simulink model "HL_control_pos_FFforce_RC_WirtualWall_Sync"  (R2020a)
settings: Solver=ode4  StartTime=0.0  StopTime=inf  FixedStep=0.001  RelTol=1e-3
libraries: xpcethercatlib x42, simulink x12, slrtlib x10, AssistOn_Gait_Lib x6
(part 2 of 3)

== system HL_control_pos_FFforce_RC_WirtualWall_Sync/Plot//Record Outputs/Left leg readings ==
  L outs : Inport
  Bus Creator : BusCreator  Inputs=2
  Bus Creator1 : BusCreator  Inputs=2
  Bus Creator2 : BusCreator  Inputs=2
  Bus Selector1 : BusSelector  OutputSignals=left.pos.y,left.vel.vy,left.force.Fy  OutputAsBus=on
  Bus Selector2 : BusSelector  OutputSignals=left.pos.theta,left.vel.omega,left.force.Tz  OutputAsBus=on
  Bus Selector4 : BusSelector  OutputSignals=left.pos.x,left.vel.vx,left.force.Fx  OutputAsBus=on
  Bus Selector5 : BusSelector  OutputSignals=lpos.lx,lvel.lvx,lFT.lFx  OutputAsBus=on
  Bus Selector6 : BusSelector  OutputSignals=lpos.ly,lvel.lvy,lFT.lFy  OutputAsBus=on
  Bus Selector7 : BusSelector  OutputSignals=lpos.ltheta,lvel.lomega,lFT.lTz  OutputAsBus=on
  "Scope " : slrtlib/Displays and Logging/Scope   scopeno=4  scopetype=Target  autostart=on  viewmode=Graphical sliding  formatstr='%15.6f'  grid=on  ylimits=80*[-1, 1]  nosamples=500  noprepostsamples=0  interleave=20  triggermode=FreeRun  triggersignal=1  trigsignalfromport=off  triggerlevel=0.0  triggerslope=Either  triggerscope=1  triggersample=0  filename=data.dat  mode=Lazy  writesize=512  autorestart=off  dynamicfilemode=off  maxwritefilesize=512*1024^2
  Scope 1 : slrtlib/Displays and Logging/Scope   scopeno=5  scopetype=Target  autostart=on  viewmode=Graphical sliding  formatstr='%15.6f'  grid=on  ylimits=80*[-1, 1]  nosamples=500  noprepostsamples=0  interleave=20  triggermode=FreeRun  triggersignal=1  trigsignalfromport=off  triggerlevel=0.0  triggerslope=Either  triggerscope=1  triggersample=0  filename=data.dat  mode=Lazy  writesize=512  autorestart=off  dynamicfilemode=off  maxwritefilesize=512*1024^2
  Scope 2 : slrtlib/Displays and Logging/Scope   scopeno=6  scopetype=Target  autostart=on  viewmode=Graphical rolling  formatstr='%15.6f'  grid=on  ylimits=pi/2*[-1, 1]  nosamples=500  noprepostsamples=0  interleave=20  triggermode=FreeRun  triggersignal=1  trigsignalfromport=off  triggerlevel=0.0  triggerslope=Either  triggerscope=1  triggersample=0  filename=data.dat  mode=Lazy  writesize=512  autorestart=off  dynamicfilemode=off  maxwritefilesize=512*1024^2
  Subsystem : Subsystem  Commented=on
  wires:
  Bus Creator/1 -> "Scope "/1
  [Ref] -> Bus Selector2/1, Bus Selector1/1, Bus Selector4/1
  Bus Creator1/1 -> Scope 1/1
  Bus Selector1/1 -> Bus Creator1/1
  Bus Selector6/1 -> Bus Creator1/2
  Bus Selector4/1 -> Bus Creator/1
  L outs/1 -> Bus Selector5/1, Bus Selector6/1, Bus Selector7/1
  Bus Creator2/1 -> Scope 2/1
  Bus Selector5/1 -> Bus Creator/2
  Bus Selector7/1 -> Bus Creator2/2
  Bus Selector2/1 -> Bus Creator2/1

== system HL_control_pos_FFforce_RC_WirtualWall_Sync/Plot//Record Outputs/Right leg readings ==
  R outs : Inport
  Bus Creator1 : BusCreator  Inputs=2
  Bus Creator2 : BusCreator  Inputs=2
  Bus Creator3 : BusCreator  Inputs=2
  Bus Selector1 : BusSelector  OutputSignals=right.pos.y,right.vel.vy,right.force.Fy  OutputAsBus=on
  Bus Selector2 : BusSelector  OutputSignals=right.pos.x,right.vel.vx,right.force.Fx  OutputAsBus=on
  Bus Selector3 : BusSelector  OutputSignals=rpos.rx,rvel.rvx,rFT.rFx  OutputAsBus=on
  Bus Selector4 : BusSelector  OutputSignals=rpos.ry,rvel.rvy,rFT.rFy  OutputAsBus=on
  Bus Selector6 : BusSelector  OutputSignals=rpos.rtheta,rvel.romega,rFT.rTz  OutputAsBus=on
  Bus Selector7 : BusSelector  OutputSignals=right.pos.theta,right.vel.omega,right.force.Tz  OutputAsBus=on
  Scope 1 : slrtlib/Displays and Logging/Scope   scopeno=2  scopetype=Target  autostart=on  viewmode=Graphical sliding  formatstr='%15.6f'  grid=on  ylimits=80*[-1, 1]  nosamples=500  noprepostsamples=0  interleave=20  triggermode=FreeRun  triggersignal=1  trigsignalfromport=off  triggerlevel=0.0  triggerslope=Either  triggerscope=1  triggersample=0  filename=rhipinc.dat  mode=Lazy  writesize=512  autorestart=off  dynamicfilemode=off  maxwritefilesize=512*1024^2
  Scope 2 : slrtlib/Displays and Logging/Scope   scopeno=1  scopetype=Target  autostart=on  viewmode=Graphical rolling  formatstr='%15.6f'  grid=on  ylimits=80*[-1, 1]  nosamples=500  noprepostsamples=0  interleave=20  triggermode=FreeRun  triggersignal=1  trigsignalfromport=off  triggerlevel=0.0  triggerslope=Either  triggerscope=1  triggersample=0  filename=rhipinc.dat  mode=Lazy  writesize=512  autorestart=off  dynamicfilemode=off  maxwritefilesize=512*1024^2
  Scope 5 : slrtlib/Displays and Logging/Scope   scopeno=3  scopetype=Target  autostart=on  viewmode=Graphical rolling  formatstr='%15.6f'  grid=on  ylimits=pi/2*[-1, 1]  nosamples=500  noprepostsamples=0  interleave=20  triggermode=FreeRun  triggersignal=1  trigsignalfromport=off  triggerlevel=0.0  triggerslope=Either  triggerscope=1  triggersample=0  filename=rhipinc.dat  mode=Lazy  writesize=512  autorestart=off  dynamicfilemode=off  maxwritefilesize=512*1024^2
  Subsystem : Subsystem  Commented=on
  wires:
  Bus Creator1/1 -> Scope 1/1
  Bus Creator2/1 -> Scope 5/1
  Bus Selector2/1 -> Bus Creator3/1
  R outs/1 -> Bus Selector3/1, Bus Selector4/1, Bus Selector6/1
  Bus Creator3/1 -> Scope 2/1
  Bus Selector4/1 -> Bus Creator1/2
  Bus Selector1/1 -> Bus Creator1/1
  Bus Selector6/1 -> Bus Creator2/2
  [Ref] -> Bus Selector7/1, Bus Selector1/1, Bus Selector2/1
  Bus Selector3/1 -> Bus Creator3/2
  Bus Selector7/1 -> Bus Creator2/1

== system HL_control_pos_FFforce_RC_WirtualWall_Sync/Right Leg/Jacobian Transpose [mN] -> [mN.mm//rad] ==
  states : Inport
  force [mN] : Inport  Port=2
  Bus Selector1 : BusSelector  OutputSignals=R disk mot.disk angle,R pos.s1s2s3,R pos.xytheta  OutputAsBus=on
  Bus to Vector : BusToVector
  S-Function : S-Function  FunctionName=RRP_Jacobian_Transpose  SFunctionModules='RRP_Jacobian_Transpose_wrapper'  SFunctionDeploymentMode=off  EnableBusSupport=off
  torque [mN.mm/rad] : Outport
  wires:
  S-Function/1 -> torque [mN.mm/rad]/1
  force [mN]/1 -> S-Function/2
  states/1 -> Bus Selector1/1
  Bus Selector1/1 -> Bus to Vector/1
  Bus to Vector/1 -> S-Function/1

== system HL_control_pos_FFforce_RC_WirtualWall_Sync/Right Leg/Position Controller -> [mN] ==
  ref pos : Inport
  ref vel : Inport  Port=2
  estimated out : Inport  Port=3
  " " : Sum
  Bus Selector : BusSelector  OutputSignals=R pos.xytheta,R vel
  D_Controller : Subsystem
  "P_Controller\t" : Subsystem
  Control Force : Outport
  wires:
  Bus Selector/2 -> D_Controller/1(Act_Vel)  "<R vel>"
  estimated out/1 -> Bus Selector/1
  "P_Controller\t"/1(P control out) -> " "/1
  Bus Selector/1 -> "P_Controller\t"/2(Act_Pos)  "<xytheta>"
  " "/1 -> Control Force/1  "Control Force"
  D_Controller/1(D control out) -> " "/2
  ref vel/1 -> D_Controller/2(Ref_vel)
  ref pos/1 -> "P_Controller\t"/1(Ref_Pos)

== system HL_control_pos_FFforce_RC_WirtualWall_Sync/Right Leg/R Actuation ==
  torque [mN.mm/rad] : Inport
  M1 Target Torque : xpcethercatlib/EtherCAT PDO Transmit   Priority=3  sig_name=M1 (MAXPOS).CST Mode.CST Outputs.TargetTorque  sig_offset=848  sig_type=int16  type_size=16  sig_dim=1  device_id=0  sample_time=0.001000
      settings: SourceProductBaseCode=XP
  M2 Target Torque : xpcethercatlib/EtherCAT PDO Transmit   Priority=3  sig_name=M2 (MAXPOS).CST Mode.CST Outputs.TargetTorque  sig_offset=992  sig_type=int16  type_size=16  sig_dim=1  device_id=0  sample_time=0.001000
      settings: SourceProductBaseCode=XP
  M3 Target Torque : xpcethercatlib/EtherCAT PDO Transmit   Priority=3  sig_name=M3 (MAXPOS).CST Mode.CST Outputs.TargetTorque  sig_offset=1104  sig_type=int16  type_size=16  sig_dim=1  device_id=0  sample_time=0.001000
      settings: SourceProductBaseCode=XP
  Target Torque : Subsystem
  wires:
  torque [mN.mm/rad]/1 -> Target Torque/1(torque)
  Target Torque/1(M1_torque) -> M1 Target Torque/1
  Target Torque/2(M2_torque) -> M2 Target Torque/1
  Target Torque/3(M3_torque) -> M3 Target Torque/1

== system HL_control_pos_FFforce_RC_WirtualWall_Sync/Right Leg/R Outputs ==
  3RRP Forward Kinematics : AssistOn_Gait_Lib/3RRP Forward Kinematics  SystemSampleTime=-1  Latency=0  AutoFrameSizeCalculation=off
  3RRP Motion Level Kinematics : AssistOn_Gait_Lib/3RRP Motion Level Kinematics  SystemSampleTime=-1  Latency=0  AutoFrameSizeCalculation=off
  Bus Creator : BusCreator  Inputs=7
  Bus Selector1 : BusSelector  OutputSignals=disk angle
  R 3RRP : AssistOn_Gait_Lib/3RRP  SystemSampleTime=-1  Latency=0  AutoFrameSizeCalculation=off
      link override 3RRP Motor Encoder Increments/M1 Position Value: sig_name=M1 (MAXPOS).CST Mode.CST Inputs.PositionActualValue  sig_offset=848  sig_type=int32  type_size=32  sig_dim=1
      link override 3RRP Motor Encoder Increments/M2 Position Value: sig_name=M2 (MAXPOS).CST Mode.CST Inputs.PositionActualValue  sig_offset=992  sig_type=int32  type_size=32  sig_dim=1
      link override 3RRP Motor Encoder Increments/M3 Position Value: sig_name=M3 (MAXPOS).CST Mode.CST Inputs.PositionActualValue  sig_offset=1104  sig_type=int32  type_size=32  sig_dim=1
      link override 3RRP Motor Torque Readings/M1 Velocity Value: sig_name=M1 (MAXPOS).CST Mode.CST Inputs.TorqueActualValue  sig_offset=912  sig_type=int16  type_size=16  sig_dim=1
      link override 3RRP Motor Torque Readings/M2 Velocity Value: sig_name=M2 (MAXPOS).CST Mode.CST Inputs.TorqueActualValue  sig_offset=1056  sig_type=int16  type_size=16  sig_dim=1
      link override 3RRP Motor Torque Readings/M3 Velocity Value: sig_name=M3 (MAXPOS).CST Mode.CST Inputs.TorqueActualValue  sig_offset=1168  sig_type=int16  type_size=16  sig_dim=1
      link override 3RRP Motor Velocity Readings/M1 Velocity Value: sig_name=M1 (MAXPOS).CST Mode.CST Inputs.Velocity Actual Value Averaged  sig_offset=880  sig_type=int32  type_size=32  sig_dim=1
      link override 3RRP Motor Velocity Readings/M2 Velocity Value: sig_name=M2 (MAXPOS).CST Mode.CST Inputs.Velocity Actual Value Averaged  sig_offset=1024  sig_type=int32  type_size=32  sig_dim=1
      link override 3RRP Motor Velocity Readings/M3 Velocity Value: sig_name=M3 (MAXPOS).CST Mode.CST Inputs.Velocity Actual Value Averaged  sig_offset=1136  sig_type=int32  type_size=32  sig_dim=1
  R Foot : Subsystem
  R Thigh : Subsystem
  R leg outs : Outport
  wires:
  R 3RRP/2 -> 3RRP Motion Level Kinematics/2, Bus Creator/5, Bus Selector1/1  "R disk mot"
  R Foot/1(Foot sens R) -> Bus Creator/7  "R_foot_sens"
  Bus Creator/1 -> R leg outs/1
  3RRP Forward Kinematics/1 -> 3RRP Motion Level Kinematics/1, Bus Creator/3  "R pos"
  Bus Selector1/1 -> 3RRP Forward Kinematics/1  "<disk angle>"
  3RRP Motion Level Kinematics/1 -> Bus Creator/4  "R vel"
  R Thigh/1(FT vals) -> Bus Creator/6  "R_thigh_FT"
  R 3RRP/1 -> Bus Creator/2  "R disk torque"
  [R_motor_T_demands] -> Bus Creator/1

== system HL_control_pos_FFforce_RC_WirtualWall_Sync/Right Leg/Velocity Sourced Compansator ==
  Velocity Disks : Inport
  Mode : Inport  Port=2
  DiskGains : Constant  Value=[1;1;3]
  MATLAB Function1 : MATLAB Function  TreatAsAtomicUnit=on
  Disk Forces : Outport
  wires:
  Velocity Disks/1 -> MATLAB Function1/1(Vel)
  Mode/1 -> MATLAB Function1/3(Mode)
  DiskGains/1 -> MATLAB Function1/2(MaxGain)
  MATLAB Function1/1(Torque) -> Disk Forces/1

== system HL_control_pos_FFforce_RC_WirtualWall_Sync/Right Leg/Virtual Wall and Syn Controller ==
  R Referance : Inport
  Virtual Wall Referance : Inport  Port=2
  L Referance : Inport  Port=3
  Synchronizer Controller : Subsystem
  Virtual Wall Controller : Subsystem
  Virtual Wall Control Signal : Outport
  Synchronizing Control Signal : Outport  Port=2
  wires:
  R Referance/1 -> Virtual Wall Controller/1(R Leg Out), Synchronizer Controller/2(R Referance)
  Virtual Wall Referance/1 -> Virtual Wall Controller/2(Referance)
  L Referance/1 -> Synchronizer Controller/1(L Referance)
  Synchronizer Controller/1(Synchronizing Control Signal) -> Synchronizing Control Signal/1
  Virtual Wall Controller/1(Virtual Wall Control Signal) -> Virtual Wall Control Signal/1

== system HL_control_pos_FFforce_RC_WirtualWall_Sync/To HMI Coord.s/L Leg ==
  pos : Inport
  vel : Inport  Port=2
  FT : Inport  Port=3
  Bus Creator : BusCreator  Inputs=3
  Bus Creator1 : BusCreator  Inputs=3
  Bus Creator2 : BusCreator  Inputs=6
  Bus to Vector : BusToVector
  Demux : Demux  Outputs=3
  Demux1 : Demux  Outputs=3
  Demux2 : Demux  Outputs=6
  FTproc : MATLAB Function  TreatAsAtomicUnit=on
  pos_vel : MATLAB Function  TreatAsAtomicUnit=on
  L pos : Outport
  L vel : Outport  Port=2
  L FT : Outport  Port=3
  wires:
  Bus Creator1/1 -> L vel/1
  Bus Creator/1 -> L pos/1
  Demux1/3 -> Bus Creator1/3  "lomega"
  Demux1/2 -> Bus Creator1/2  "lvy"
  Demux1/1 -> Bus Creator1/1  "lvx"
  Demux/2 -> Bus Creator/2  "ly"
  Demux/1 -> Bus Creator/1  "lx"
  pos/1 -> pos_vel/1("pos ")
  pos_vel/2(vel) -> Demux1/1  "L vel"
  pos_vel/1(pos) -> Demux/1  "L pos"
  vel/1 -> pos_vel/2("vel ")
  Bus Creator2/1 -> L FT/1  "l FT"
  FT/1 -> Bus to Vector/1
  Demux/3 -> FTproc/1(theta), Bus Creator/3  "ltheta"
  Demux2/1 -> Bus Creator2/1  "lFx"
  Demux2/2 -> Bus Creator2/2  "lFy"
  Demux2/3 -> Bus Creator2/3  "lFz"
  Bus to Vector/1 -> FTproc/2("FT ")
  Demux2/6 -> Bus Creator2/6  "lTz"
  Demux2/4 -> Bus Creator2/4  "lTx"
  Demux2/5 -> Bus Creator2/5  "lTy"
  FTproc/1(FT) -> Demux2/1

== system HL_control_pos_FFforce_RC_WirtualWall_Sync/To HMI Coord.s/R Leg ==
  pos : Inport
  vel : Inport  Port=2
  FT : Inport  Port=3
  Bus Creator : BusCreator  Inputs=3
  Bus Creator1 : BusCreator  Inputs=3
  Bus Creator2 : BusCreator  Inputs=6
  Bus to Vector : BusToVector
  Demux : Demux  Outputs=3
  Demux1 : Demux  Outputs=3
  Demux2 : Demux  Outputs=6
  FTproc : MATLAB Function  TreatAsAtomicUnit=on
  pos_vel : MATLAB Function  TreatAsAtomicUnit=on
  R pos : Outport
  R vel : Outport  Port=2
  R FT : Outport  Port=3
  wires:
  vel/1 -> pos_vel/2("vel ")
  pos_vel/1(pos) -> Demux/1  "R pos"
  pos_vel/2(vel) -> Demux1/1  "R vel"
  pos/1 -> pos_vel/1("pos ")
  Demux/1 -> Bus Creator/1  "rx"
  Demux/2 -> Bus Creator/2  "ry"
  Demux/3 -> FTproc/1(theta), Bus Creator/3  "rtheta"
  Demux1/1 -> Bus Creator1/1  "rvx"
  Demux1/2 -> Bus Creator1/2  "rvy"
  Demux1/3 -> Bus Creator1/3  "romega"
  Bus Creator/1 -> R pos/1  "rpos"
  Bus Creator1/1 -> R vel/1  "rvel"
  Bus Creator2/1 -> R FT/1  "rFT"
  FTproc/1(FT) -> Demux2/1
  Demux2/1 -> Bus Creator2/1  "rFx"
  Demux2/2 -> Bus Creator2/2  "rFy"
  Demux2/3 -> Bus Creator2/3  "rFz"
  Demux2/4 -> Bus Creator2/4  "rTx"
  Demux2/5 -> Bus Creator2/5  "rTy"
  Demux2/6 -> Bus Creator2/6  "rTz"
  FT/1 -> Bus to Vector/1
  Bus to Vector/1 -> FTproc/2("FT ")

== system HL_control_pos_FFforce_RC_WirtualWall_Sync/Left Leg/L Actuation/Target Torque ==
  torque : Inport
  Data Type Conversion2 : DataTypeConversion  OutDataTypeStr=int16
  Demux1 : Demux  Outputs=3
  INT16_Limit : Saturate  UpperLimit=[2^15-1 2^15-1 2^15-1]  LowerLimit=[-2^15 -2^15 -2^15]
  Torque Saturation : Subsystem
  capstan_ratio : Gain  Gain=1/30
  direction : Gain  Gain=-1  OutDataTypeStr=double
  per 1000 of rated torque [mN.m] : Gain  Gain=1000/(5*123)  OutDataTypeStr=double
  M1_torque : Outport  VectorParamsAs1DForOutWhenUnconnected=off
  M2_torque : Outport  Port=2  VectorParamsAs1DForOutWhenUnconnected=off
  M3_torque : Outport  Port=3  VectorParamsAs1DForOutWhenUnconnected=off
  tag scope: L_motor_T_demands=global
  wires:
  Torque Saturation/1(adjusted torque) -> per 1000 of rated torque [mN.m]/1  "Torques"
  Demux1/3 -> M3_torque/1
  Demux1/2 -> M2_torque/1
  Demux1/1 -> M1_torque/1
  per 1000 of rated torque [mN.m]/1 -> INT16_Limit/1
  INT16_Limit/1 -> Data Type Conversion2/1
  Data Type Conversion2/1 -> Demux1/1
  capstan_ratio/1 -> direction/1
  torque/1 -> capstan_ratio/1
  direction/1 -> Torque Saturation/1(demanded torque), [L_motor_T_demands]  "L Motor Torques"

== system HL_control_pos_FFforce_RC_WirtualWall_Sync/Left Leg/L Outputs/L Foot ==
  IsoM_M1_Position_Value : xpcethercatlib/EtherCAT PDO Receive  Priority=2  sig_name=AIO (EL3008).AI Standard Channel 8.Value  sig_offset=2128  sig_type=int16  type_size=16  sig_dim=1  device_id=0  sample_time=0.001000
      settings: SourceProductBaseCode=XP
  V : Gain  Gain=20/65535
  from int16 : DataTypeConversion  OutDataTypeStr=double
  Foot sens L : Outport
  wires:
  from int16/1 -> V/1  "Analog value [double]"
  V/1 -> Foot sens L/1  "Foot pressure [V]"
  IsoM_M1_Position_Value/1 -> from int16/1  "Analog value [16-bit int]"

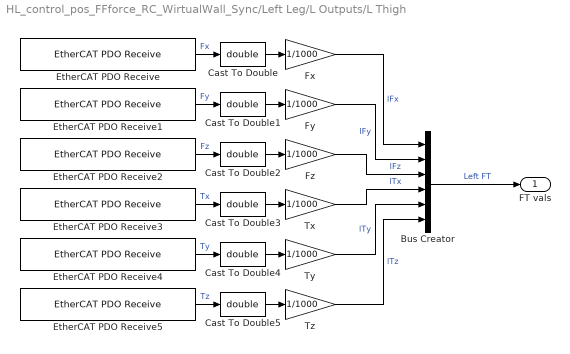
== system HL_control_pos_FFforce_RC_WirtualWall_Sync/Left Leg/L Outputs/L Thigh ==
  Bus Creator : BusCreator  Inputs=6
  Cast To Double{,1..5} (6 alike) : DataTypeConversion  OutDataTypeStr=double
  EtherCAT PDO Receive : xpcethercatlib/EtherCAT PDO Receive  Priority=2  sig_name=Left F/T.Reading Data.Fx/Gage0  sig_offset=1536  sig_type=int32  type_size=32  sig_dim=1  device_id=0  sample_time=0.001000
      settings: SourceProductBaseCode=XP
  EtherCAT PDO Receive1 : xpcethercatlib/EtherCAT PDO Receive  Priority=2  sig_name=Left F/T.Reading Data.Fy/Gage1  sig_offset=1568  sig_type=int32  type_size=32  sig_dim=1  device_id=0  sample_time=0.001000
      settings: SourceProductBaseCode=XP
  EtherCAT PDO Receive2 : xpcethercatlib/EtherCAT PDO Receive  Priority=2  sig_name=Left F/T.Reading Data.Fz/Gage2  sig_offset=1600  sig_type=int32  type_size=32  sig_dim=1  device_id=0  sample_time=0.001000
      settings: SourceProductBaseCode=XP
  EtherCAT PDO Receive3 : xpcethercatlib/EtherCAT PDO Receive  Priority=2  sig_name=Left F/T.Reading Data.Tx/Gage3  sig_offset=1632  sig_type=int32  type_size=32  sig_dim=1  device_id=0  sample_time=0.001000
      settings: SourceProductBaseCode=XP
  EtherCAT PDO Receive4 : xpcethercatlib/EtherCAT PDO Receive  Priority=2  sig_name=Left F/T.Reading Data.Ty/Gage4  sig_offset=1664  sig_type=int32  type_size=32  sig_dim=1  device_id=0  sample_time=0.001000
      settings: SourceProductBaseCode=XP
  EtherCAT PDO Receive5 : xpcethercatlib/EtherCAT PDO Receive  Priority=2  sig_name=Left F/T.Reading Data.Tz/Gage5  sig_offset=1696  sig_type=int32  type_size=32  sig_dim=1  device_id=0  sample_time=0.001000
      settings: SourceProductBaseCode=XP
  Fx : Gain  Gain=1/1000  OutDataTypeStr=double
  Fy : Gain  Gain=1/1000  OutDataTypeStr=double
  Fz : Gain  Gain=1/1000  OutDataTypeStr=double
  Tx : Gain  Gain=1/1000  OutDataTypeStr=double
  Ty : Gain  Gain=1/1000  OutDataTypeStr=double
  Tz : Gain  Gain=1/1000  OutDataTypeStr=double
  FT vals : Outport
  wires:
  Tx/1 -> Bus Creator/4  "lTx"
  Fx/1 -> Bus Creator/1  "lFx"
  EtherCAT PDO Receive/1 -> Cast To Double/1  "Fx"
  Ty/1 -> Bus Creator/5  "lTy"
  EtherCAT PDO Receive5/1 -> Cast To Double5/1  "Tz"
  Tz/1 -> Bus Creator/6  "lTz"
  EtherCAT PDO Receive2/1 -> Cast To Double2/1  "Fz"
  EtherCAT PDO Receive4/1 -> Cast To Double4/1  "Ty"
  EtherCAT PDO Receive3/1 -> Cast To Double3/1  "Tx"
  Bus Creator/1 -> FT vals/1  "Left FT"
  Fy/1 -> Bus Creator/2  "lFy"
  Fz/1 -> Bus Creator/3  "lFz"
  EtherCAT PDO Receive1/1 -> Cast To Double1/1  "Fy"
  Cast To Double/1 -> Fx/1
  Cast To Double1/1 -> Fy/1
  Cast To Double2/1 -> Fz/1
  Cast To Double3/1 -> Tx/1
  Cast To Double4/1 -> Ty/1
  Cast To Double5/1 -> Tz/1

== system HL_control_pos_FFforce_RC_WirtualWall_Sync/Left Leg/Position Controller -> [mN]/D_Controller ==
  Act_Vel : Inport
  Ref_vel : Inport  Port=2
  D_Gain : DataStoreRead  DataStoreName=Dgain
  D_Gain_Multiplier : Product
  Error_Vel : Sum  Inputs=+-
  Gain : Gain  Gain=[0.04; 0.04; 30]
  D control out : Outport  VectorParamsAs1DForOutWhenUnconnected=off
  wires:
  Error_Vel/1 -> Gain/1
  D_Gain_Multiplier/1 -> D control out/1
  Ref_vel/1 -> Error_Vel/1
  D_Gain/1 -> D_Gain_Multiplier/1
  Act_Vel/1 -> Error_Vel/2
  Gain/1 -> D_Gain_Multiplier/2

== system HL_control_pos_FFforce_RC_WirtualWall_Sync/Left Leg/Position Controller -> [mN]/P_Controller	 ==
  Ref_Pos : Inport
  Act_Pos : Inport  Port=2
  Add : Sum  Inputs=+-
  Gain : Gain  Gain=[3; 3; 7000]
  P_Gain : DataStoreRead  DataStoreName=Pgain
  P_Gain_Multiplier : Product
  P control out : Outport  VectorParamsAs1DForOutWhenUnconnected=off
  wires:
  Ref_Pos/1 -> Add/1
  P_Gain/1 -> P_Gain_Multiplier/1
  Add/1 -> Gain/1
  Gain/1 -> P_Gain_Multiplier/2
  P_Gain_Multiplier/1 -> P control out/1
  Act_Pos/1 -> Add/2

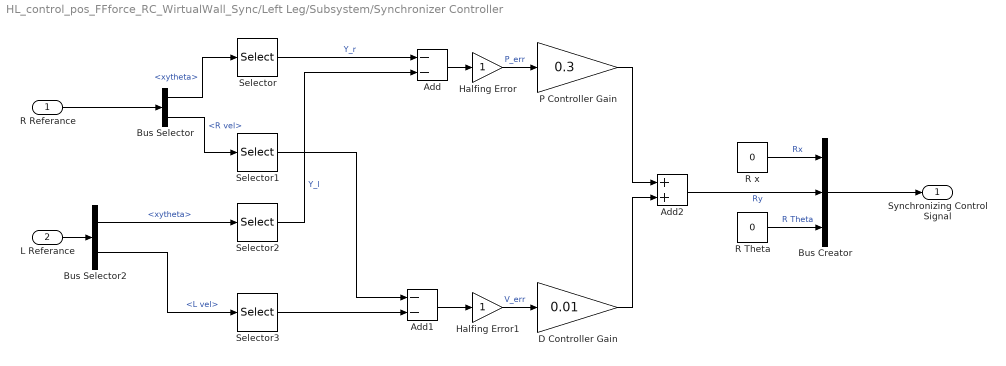
== system HL_control_pos_FFforce_RC_WirtualWall_Sync/Left Leg/Subsystem/Synchronizer Controller ==
  R Referance : Inport
  L Referance : Inport  Port=2
  " P Controller Gain" : Gain  Gain=0.3
  Add : Sum  Inputs=--
  Add1 : Sum  Inputs=--
  Add2 : Sum
  Bus Creator : BusCreator  Inputs=3
  Bus Selector : BusSelector  OutputSignals=xytheta,R vel
  Bus Selector2 : BusSelector  OutputSignals=L pos.xytheta,L vel
  D Controller Gain : Gain  Gain=0.01
  Halfing Error : Gain
  Halfing Error1 : Gain
  R Theta : Constant  Value=0
  "R x " : Constant  Value=0
  Selector{,1..3} (4 alike) : Selector  InputPortWidth=3  IndexOptions=Index vector (dialog)  Indices=[2]  OutputSizes=1
  Synchronizing Control Signal : Outport
  wires:
  R Referance/1 -> Bus Selector/1
  Bus Selector/2 -> Selector1/1  "<R vel>"
  Selector2/1 -> Add/2  "Y_l"
  Selector1/1 -> Add1/1
  Selector3/1 -> Add1/2
  Add/1 -> Halfing Error/1
  Halfing Error/1 -> " P Controller Gain"/1  "P_err"
  Halfing Error1/1 -> D Controller Gain/1  "V_err"
  Add1/1 -> Halfing Error1/1
  " P Controller Gain"/1 -> Add2/1
  D Controller Gain/1 -> Add2/2
  Add2/1 -> Bus Creator/2  "Ry"
  "R x "/1 -> Bus Creator/1  "Rx"
  R Theta/1 -> Bus Creator/3  "R Theta"
  Bus Creator/1 -> Synchronizing Control Signal/1
  L Referance/1 -> Bus Selector2/1
  Bus Selector2/1 -> Selector2/1  "<xytheta>"
  Bus Selector2/2 -> Selector3/1  "<L vel>"
  Bus Selector/1 -> Selector/1  "<xytheta>"
  Selector/1 -> Add/1  "Y_r"

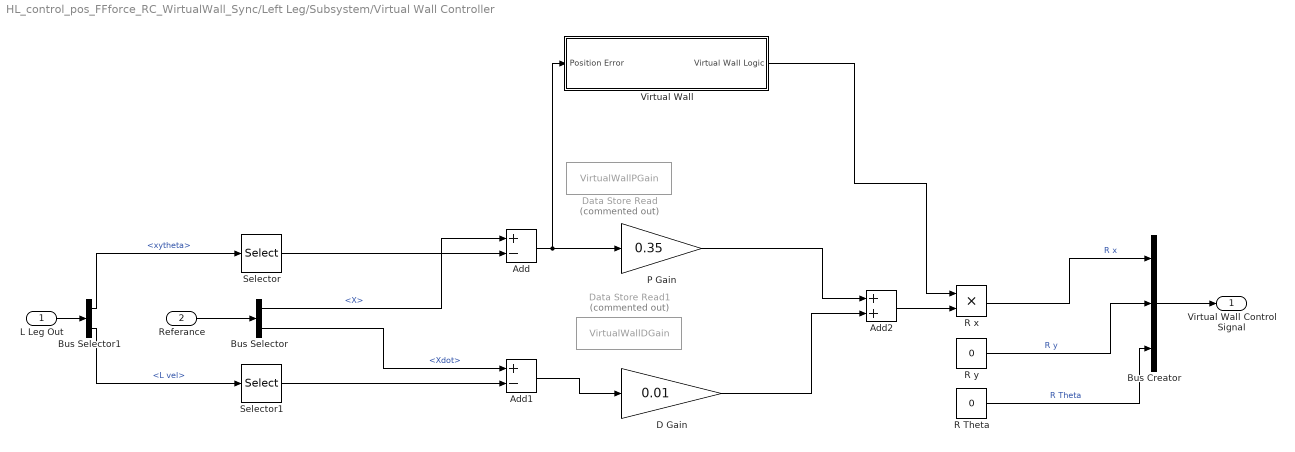
== system HL_control_pos_FFforce_RC_WirtualWall_Sync/Left Leg/Subsystem/Virtual Wall Controller ==
  L Leg Out : Inport
  Referance : Inport  Port=2
  Add : Sum  Inputs=+-
  Add1 : Sum  Inputs=+-
  Add2 : Sum
  Bus Creator : BusCreator  Inputs=3
  Bus Selector : BusSelector  OutputSignals=X,Xdot
  Bus Selector1 : BusSelector  OutputSignals=L pos.xytheta,L vel
  D Gain : Gain  Gain=0.01
  Data Store Read : DataStoreRead  Commented=on  DataStoreName=VirtualWallPGain
  Data Store Read1 : DataStoreRead  Commented=on  DataStoreName=VirtualWallDGain
  P Gain : Gain  Gain=0.35
  R Theta : Constant  Value=0
  R x : Product
  R y : Constant  Value=0
  Selector : Selector  InputPortWidth=3  IndexOptions=Index vector (dialog)  Indices=[1]  OutputSizes=1
  Selector1 : Selector  InputPortWidth=3  IndexOptions=Index vector (dialog)  Indices=[1]  OutputSizes=1
  Virtual Wall : Subsystem
  Virtual Wall Control Signal : Outport
  wires:
  Referance/1 -> Bus Selector/1
  Add1/1 -> D Gain/1
  Virtual Wall/1(Virtual Wall Logic) -> R x/1
  Add/1 -> Virtual Wall/1(Position Error), P Gain/1
  P Gain/1 -> Add2/1
  D Gain/1 -> Add2/2
  Add2/1 -> R x/2
  R x/1 -> Bus Creator/1  "R x"
  Bus Creator/1 -> Virtual Wall Control Signal/1
  R y/1 -> Bus Creator/2  "R y"
  R Theta/1 -> Bus Creator/3  "R Theta"
  Bus Selector/2 -> Add1/1  "<Xdot>"
  Bus Selector/1 -> Add/1  "<X>"
  Selector/1 -> Add/2
  Selector1/1 -> Add1/2
  Bus Selector1/1 -> Selector/1  "<xytheta>"
  Bus Selector1/2 -> Selector1/1  "<L vel>"
  L Leg Out/1 -> Bus Selector1/1

== system HL_control_pos_FFforce_RC_WirtualWall_Sync/Plot//Record Outputs/Left leg readings/Subsystem ==
  rot : Inport
  Bus Creator3 : BusCreator  Inputs=3
  Bus Selector5 : BusSelector  OutputSignals=left.pos.theta,left.vel.omega,left.force.Tz
  Divide : Product  Inputs=*/
  Torque Limit : DataStoreRead  DataStoreName=Torque_scale
  scaled : Outport
  wires:
  Bus Creator3/1 -> scaled/1
  Bus Selector5/1 -> Bus Creator3/1  "<theta>"
  Divide/1 -> Bus Creator3/3  "Tz"
  Torque Limit/1 -> Divide/2
  Bus Selector5/3 -> Divide/1  "<Tz>"
  Bus Selector5/2 -> Bus Creator3/2  "<omega>"
  rot/1 -> Bus Selector5/1

== system HL_control_pos_FFforce_RC_WirtualWall_Sync/Plot//Record Outputs/Right leg readings/Subsystem ==
  rot : Inport
  Bus Creator3 : BusCreator  Inputs=3
  Bus Selector5 : BusSelector  OutputSignals=right.pos.theta,right.vel.omega,right.force.Tz
  Divide : Product  Inputs=*/
  Torque Limit : DataStoreRead  DataStoreName=Torque_scale
  scaled : Outport
  wires:
  Bus Creator3/1 -> scaled/1
  Bus Selector5/1 -> Bus Creator3/1  "<theta>"
  Divide/1 -> Bus Creator3/3  "Tz"
  Torque Limit/1 -> Divide/2
  Bus Selector5/3 -> Divide/1  "<Tz>"
  Bus Selector5/2 -> Bus Creator3/2  "<omega>"
  rot/1 -> Bus Selector5/1

== system HL_control_pos_FFforce_RC_WirtualWall_Sync/Right Leg/Position Controller -> [mN]/D_Controller ==
  Act_Vel : Inport
  Ref_vel : Inport  Port=2
  D_Gain : DataStoreRead  DataStoreName=Dgain
  D_Gain_Multiplier : Product
  Error_Vel : Sum  Inputs=+-
  Gain : Gain  Gain=[0.04; 0.04; 30]
  D control out : Outport  VectorParamsAs1DForOutWhenUnconnected=off
  wires:
  Error_Vel/1 -> Gain/1
  D_Gain_Multiplier/1 -> D control out/1
  Ref_vel/1 -> Error_Vel/1
  D_Gain/1 -> D_Gain_Multiplier/1
  Act_Vel/1 -> Error_Vel/2
  Gain/1 -> D_Gain_Multiplier/2

== system HL_control_pos_FFforce_RC_WirtualWall_Sync/Right Leg/Position Controller -> [mN]/P_Controller	 ==
  Ref_Pos : Inport
  Act_Pos : Inport  Port=2
  Add : Sum  Inputs=+-
  Gain : Gain  Gain=[3; 3; 7000]
  P_Gain : DataStoreRead  DataStoreName=Pgain
  P_Gain_Multiplier : Product
  P control out : Outport  VectorParamsAs1DForOutWhenUnconnected=off
  wires:
  Ref_Pos/1 -> Add/1
  P_Gain/1 -> P_Gain_Multiplier/1
  Add/1 -> Gain/1
  Gain/1 -> P_Gain_Multiplier/2
  P_Gain_Multiplier/1 -> P control out/1
  Act_Pos/1 -> Add/2

== system HL_control_pos_FFforce_RC_WirtualWall_Sync/Right Leg/R Actuation/Target Torque ==
  torque : Inport
  Data Type Conversion2 : DataTypeConversion  OutDataTypeStr=int16
  Demux1 : Demux  Outputs=3
  INT16_Limit : Saturate  UpperLimit=[2^15-1 2^15-1 2^15-1]  LowerLimit=[-2^15 -2^15 -2^15]
  Torque Saturation : Subsystem
  capstan_ratio : Gain  Gain=1/30
  direction : Gain  Gain=-1  OutDataTypeStr=double
  per 1000 of rated torque [mN.m] : Gain  Gain=1000/(5*123)  OutDataTypeStr=double
  M1_torque : Outport  VectorParamsAs1DForOutWhenUnconnected=off
  M2_torque : Outport  Port=2  VectorParamsAs1DForOutWhenUnconnected=off
  M3_torque : Outport  Port=3  VectorParamsAs1DForOutWhenUnconnected=off
  tag scope: R_motor_T_demands=global
  wires:
  direction/1 -> [R_motor_T_demands], Torque Saturation/1(demanded torque)  "R Motor Torques"
  torque/1 -> capstan_ratio/1
  capstan_ratio/1 -> direction/1
  Data Type Conversion2/1 -> Demux1/1
  INT16_Limit/1 -> Data Type Conversion2/1
  per 1000 of rated torque [mN.m]/1 -> INT16_Limit/1
  Demux1/1 -> M1_torque/1
  Demux1/2 -> M2_torque/1
  Demux1/3 -> M3_torque/1
  Torque Saturation/1(adjusted torque) -> per 1000 of rated torque [mN.m]/1  "Torques"

== system HL_control_pos_FFforce_RC_WirtualWall_Sync/Right Leg/R Outputs/R Foot ==
  IsoM_M1_Position_Value : xpcethercatlib/EtherCAT PDO Receive  Priority=2  sig_name=AIO (EL3008).AI Standard Channel 7.Value  sig_offset=2096  sig_type=int16  type_size=16  sig_dim=1  device_id=0  sample_time=0.001000
      settings: SourceProductBaseCode=XP
  V : Gain  Gain=20/65535
  from int16 : DataTypeConversion  OutDataTypeStr=double
  Foot sens R : Outport
  wires:
  IsoM_M1_Position_Value/1 -> from int16/1  "Analog value [16-bit int]"
  V/1 -> Foot sens R/1  "Foot pressure [V]"
  from int16/1 -> V/1  "Analog value [double]"

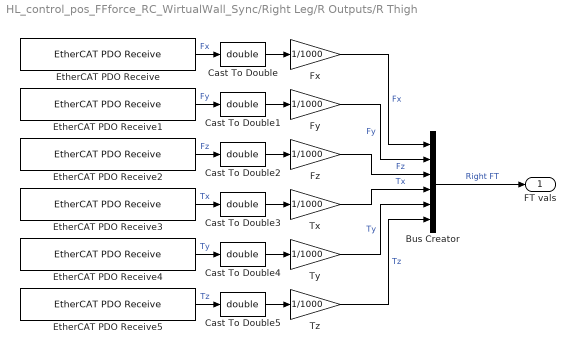
== system HL_control_pos_FFforce_RC_WirtualWall_Sync/Right Leg/R Outputs/R Thigh ==
  Bus Creator : BusCreator  Inputs=6
  Cast To Double{,1..5} (6 alike) : DataTypeConversion  OutDataTypeStr=double
  EtherCAT PDO Receive : xpcethercatlib/EtherCAT PDO Receive  Priority=2  sig_name=Right F/T.Reading Data.Fx/Gage0  sig_offset=576  sig_type=int32  type_size=32  sig_dim=1  device_id=0  sample_time=0.001000
      settings: SourceProductBaseCode=XP
  EtherCAT PDO Receive1 : xpcethercatlib/EtherCAT PDO Receive  Priority=2  sig_name=Right F/T.Reading Data.Fy/Gage1  sig_offset=608  sig_type=int32  type_size=32  sig_dim=1  device_id=0  sample_time=0.001000
      settings: SourceProductBaseCode=XP
  EtherCAT PDO Receive2 : xpcethercatlib/EtherCAT PDO Receive  Priority=2  sig_name=Right F/T.Reading Data.Fz/Gage2  sig_offset=640  sig_type=int32  type_size=32  sig_dim=1  device_id=0  sample_time=0.001000
      settings: SourceProductBaseCode=XP
  EtherCAT PDO Receive3 : xpcethercatlib/EtherCAT PDO Receive  Priority=2  sig_name=Right F/T.Reading Data.Tx/Gage3  sig_offset=672  sig_type=int32  type_size=32  sig_dim=1  device_id=0  sample_time=0.001000
      settings: SourceProductBaseCode=XP
  EtherCAT PDO Receive4 : xpcethercatlib/EtherCAT PDO Receive  Priority=2  sig_name=Right F/T.Reading Data.Ty/Gage4  sig_offset=704  sig_type=int32  type_size=32  sig_dim=1  device_id=0  sample_time=0.001000
      settings: SourceProductBaseCode=XP
  EtherCAT PDO Receive5 : xpcethercatlib/EtherCAT PDO Receive  Priority=2  sig_name=Right F/T.Reading Data.Tz/Gage5  sig_offset=736  sig_type=int32  type_size=32  sig_dim=1  device_id=0  sample_time=0.001000
      settings: SourceProductBaseCode=XP
  Fx : Gain  Gain=1/1000  OutDataTypeStr=double
  Fy : Gain  Gain=1/1000  OutDataTypeStr=double
  Fz : Gain  Gain=1/1000  OutDataTypeStr=double
  Tx : Gain  Gain=1/1000  OutDataTypeStr=double
  Ty : Gain  Gain=1/1000  OutDataTypeStr=double
  Tz : Gain  Gain=1/1000  OutDataTypeStr=double
  FT vals : Outport
  wires:
  Bus Creator/1 -> FT vals/1  "Right FT"
  Fy/1 -> Bus Creator/2  "Fy"
  Fz/1 -> Bus Creator/3  "Fz"
  Tx/1 -> Bus Creator/4  "Tx"
  Ty/1 -> Bus Creator/5  "Ty"
  Tz/1 -> Bus Creator/6  "Tz"
  Fx/1 -> Bus Creator/1  "Fx"
  EtherCAT PDO Receive/1 -> Cast To Double/1  "Fx"
  EtherCAT PDO Receive1/1 -> Cast To Double1/1  "Fy"
  EtherCAT PDO Receive2/1 -> Cast To Double2/1  "Fz"
  EtherCAT PDO Receive3/1 -> Cast To Double3/1  "Tx"
  EtherCAT PDO Receive4/1 -> Cast To Double4/1  "Ty"
  EtherCAT PDO Receive5/1 -> Cast To Double5/1  "Tz"
  Cast To Double/1 -> Fx/1
  Cast To Double1/1 -> Fy/1
  Cast To Double3/1 -> Tx/1
  Cast To Double4/1 -> Ty/1
  Cast To Double2/1 -> Fz/1
  Cast To Double5/1 -> Tz/1

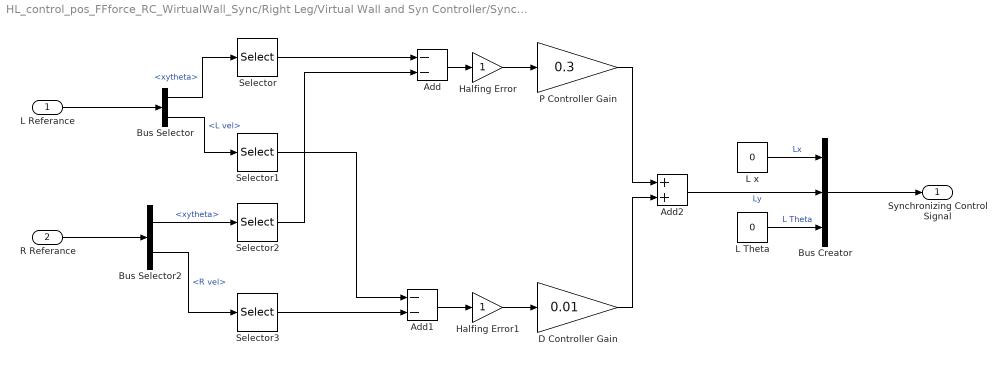
== system HL_control_pos_FFforce_RC_WirtualWall_Sync/Right Leg/Virtual Wall and Syn Controller/Synchronizer Controller ==
  L Referance : Inport
  R Referance : Inport  Port=2
  " P Controller Gain" : Gain  Gain=0.3
  Add : Sum  Inputs=--
  Add1 : Sum  Inputs=--
  Add2 : Sum
  Bus Creator : BusCreator  Inputs=3
  Bus Selector : BusSelector  OutputSignals=xytheta,L vel
  Bus Selector2 : BusSelector  OutputSignals=R pos.xytheta,R vel
  D Controller Gain : Gain  Gain=0.01
  Halfing Error : Gain
  Halfing Error1 : Gain
  L Theta : Constant  Value=0
  "L x " : Constant  Value=0
  Selector{,1..3} (4 alike) : Selector  InputPortWidth=3  IndexOptions=Index vector (dialog)  Indices=[2]  OutputSizes=1
  Synchronizing Control Signal : Outport
  wires:
  L Referance/1 -> Bus Selector/1
  Bus Selector/2 -> Selector1/1  "<L vel>"
  Selector/1 -> Add/1
  Selector2/1 -> Add/2
  Selector1/1 -> Add1/1
  Selector3/1 -> Add1/2
  Add/1 -> Halfing Error/1
  Halfing Error/1 -> " P Controller Gain"/1
  Halfing Error1/1 -> D Controller Gain/1
  Add1/1 -> Halfing Error1/1
  " P Controller Gain"/1 -> Add2/1
  D Controller Gain/1 -> Add2/2
  Add2/1 -> Bus Creator/2  "Ly"
  "L x "/1 -> Bus Creator/1  "Lx"
  L Theta/1 -> Bus Creator/3  "L Theta"
  Bus Creator/1 -> Synchronizing Control Signal/1
  R Referance/1 -> Bus Selector2/1
  Bus Selector2/1 -> Selector2/1  "<xytheta>"
  Bus Selector2/2 -> Selector3/1  "<R vel>"
  Bus Selector/1 -> Selector/1  "<xytheta>"

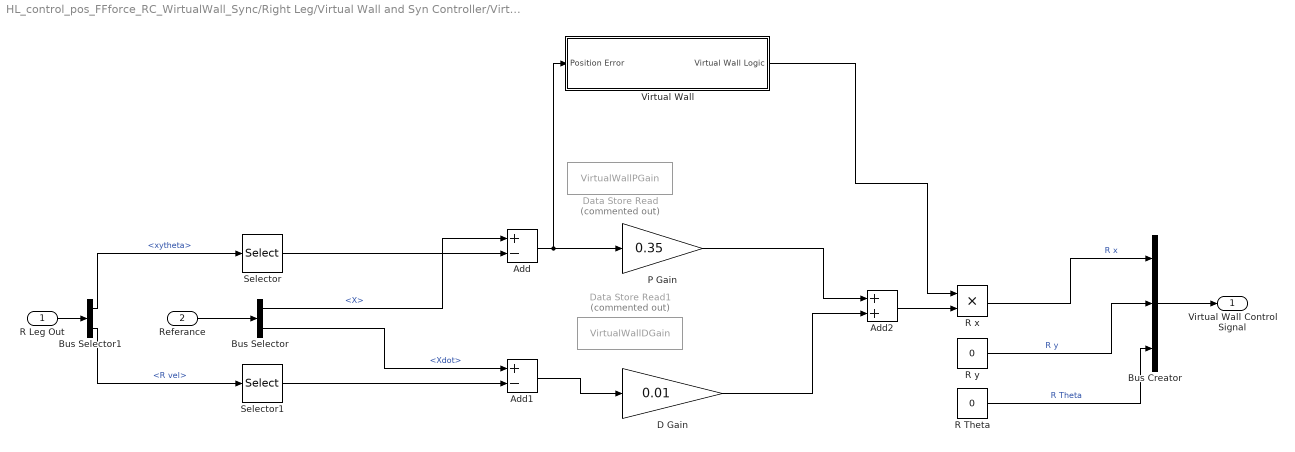
== system HL_control_pos_FFforce_RC_WirtualWall_Sync/Right Leg/Virtual Wall and Syn Controller/Virtual Wall Controller ==
  R Leg Out : Inport
  Referance : Inport  Port=2
  Add : Sum  Inputs=+-
  Add1 : Sum  Inputs=+-
  Add2 : Sum
  Bus Creator : BusCreator  Inputs=3
  Bus Selector : BusSelector  OutputSignals=X,Xdot
  Bus Selector1 : BusSelector  OutputSignals=R pos.xytheta,R vel
  D Gain : Gain  Gain=0.01
  Data Store Read : DataStoreRead  Commented=on  DataStoreName=VirtualWallPGain
  Data Store Read1 : DataStoreRead  Commented=on  DataStoreName=VirtualWallDGain
  P Gain : Gain  Gain=0.35
  R Theta : Constant  Value=0
  R x : Product
  R y : Constant  Value=0
  Selector : Selector  InputPortWidth=3  IndexOptions=Index vector (dialog)  Indices=[1]  OutputSizes=1
  Selector1 : Selector  InputPortWidth=3  IndexOptions=Index vector (dialog)  Indices=[1]  OutputSizes=1
  Virtual Wall : Subsystem
  Virtual Wall Control Signal : Outport
  wires:
  Referance/1 -> Bus Selector/1
  Add1/1 -> D Gain/1
  Virtual Wall/1(Virtual Wall Logic) -> R x/1
  Add/1 -> Virtual Wall/1(Position Error), P Gain/1
  P Gain/1 -> Add2/1
  D Gain/1 -> Add2/2
  Add2/1 -> R x/2
  R x/1 -> Bus Creator/1  "R x"
  Bus Creator/1 -> Virtual Wall Control Signal/1
  R y/1 -> Bus Creator/2  "R y"
  R Theta/1 -> Bus Creator/3  "R Theta"
  Bus Selector/2 -> Add1/1  "<Xdot>"
  Bus Selector/1 -> Add/1  "<X>"
  Selector/1 -> Add/2
  Selector1/1 -> Add1/2
  Bus Selector1/1 -> Selector/1  "<xytheta>"
  Bus Selector1/2 -> Selector1/1  "<R vel>"
  R Leg Out/1 -> Bus Selector1/1

== system HL_control_pos_FFforce_RC_WirtualWall_Sync/Left Leg/L Actuation/Target Torque/Torque Saturation ==
  demanded torque : Inport
  Demux2 : Demux  Outputs=3
  Mux1 : Mux  Inputs=3
  Saturation Dynamic : simulink/Discontinuities/Saturation Dynamic  OutMin=[]  OutMax=[]  OutDataTypeStr=Inherit: Same as second input  OutDataType=fixdt(1, 16)  OutScaling=2^-10  RndMeth=Simplest  DoSatur=off
  Saturation Dynamic1 : simulink/Discontinuities/Saturation Dynamic  OutMin=[]  OutMax=[]  OutDataTypeStr=Inherit: Same as second input  OutDataType=fixdt(1, 16)  OutScaling=2^-10  RndMeth=Simplest  DoSatur=off
  Saturation Dynamic2 : simulink/Discontinuities/Saturation Dynamic  OutMin=[]  OutMax=[]  OutDataTypeStr=Inherit: Same as second input  OutDataType=fixdt(1, 16)  OutScaling=2^-10  RndMeth=Simplest  DoSatur=off
  Torque Limit : DataStoreRead  DataStoreName=Motor_torque_limit
  negative : Gain  Gain=-1  OutDataTypeStr=double
  adjusted torque : Outport
  wires:
  demanded torque/1 -> Demux2/1
  Demux2/3 -> Saturation Dynamic2/2
  Saturation Dynamic/1 -> Mux1/1
  Saturation Dynamic1/1 -> Mux1/2
  negative/1 -> Saturation Dynamic1/3, Saturation Dynamic2/3, Saturation Dynamic/3
  Saturation Dynamic2/1 -> Mux1/3
  Mux1/1 -> adjusted torque/1
  Demux2/1 -> Saturation Dynamic/2
  Demux2/2 -> Saturation Dynamic1/2
  Torque Limit/1 -> negative/1, Saturation Dynamic2/1, Saturation Dynamic1/1, Saturation Dynamic/1

== system HL_control_pos_FFforce_RC_WirtualWall_Sync/Left Leg/Subsystem/Virtual Wall Controller/Virtual Wall ==
  Position Error : Inport
  Abs : Abs
  Constant : Constant  Value=0
  Switch : Switch  Criteria=u2 > Threshold  Threshold=5
  Virtual Wall Logic : Outport
  wires:
  Position Error/1 -> Abs/1
  Constant/1 -> Switch/3
  Abs/1 -> Switch/1, Switch/2
  Switch/1 -> Virtual Wall Logic/1

== system HL_control_pos_FFforce_RC_WirtualWall_Sync/Right Leg/R Actuation/Target Torque/Torque Saturation ==
  demanded torque : Inport
  Demux2 : Demux  Outputs=3
  Mux1 : Mux  Inputs=3
  Saturation Dynamic : simulink/Discontinuities/Saturation Dynamic  OutMin=[]  OutMax=[]  OutDataTypeStr=Inherit: Same as second input  OutDataType=fixdt(1, 16)  OutScaling=2^-10  RndMeth=Simplest  DoSatur=off
  Saturation Dynamic1 : simulink/Discontinuities/Saturation Dynamic  OutMin=[]  OutMax=[]  OutDataTypeStr=Inherit: Same as second input  OutDataType=fixdt(1, 16)  OutScaling=2^-10  RndMeth=Simplest  DoSatur=off
  Saturation Dynamic2 : simulink/Discontinuities/Saturation Dynamic  OutMin=[]  OutMax=[]  OutDataTypeStr=Inherit: Same as second input  OutDataType=fixdt(1, 16)  OutScaling=2^-10  RndMeth=Simplest  DoSatur=off
  Torque Limit : DataStoreRead  DataStoreName=Motor_torque_limit
  negative : Gain  Gain=-1  OutDataTypeStr=double
  adjusted torque : Outport
  wires:
  Torque Limit/1 -> Saturation Dynamic/1, Saturation Dynamic1/1, Saturation Dynamic2/1, negative/1
  Demux2/2 -> Saturation Dynamic1/2
  Demux2/1 -> Saturation Dynamic/2
  Mux1/1 -> adjusted torque/1
  Saturation Dynamic2/1 -> Mux1/3
  negative/1 -> Saturation Dynamic/3, Saturation Dynamic2/3, Saturation Dynamic1/3
  Saturation Dynamic1/1 -> Mux1/2
  Saturation Dynamic/1 -> Mux1/1
  Demux2/3 -> Saturation Dynamic2/2
  demanded torque/1 -> Demux2/1

== system HL_control_pos_FFforce_RC_WirtualWall_Sync/Right Leg/Virtual Wall and Syn Controller/Virtual Wall Controller/Virtual Wall ==
  Position Error : Inport
  Abs : Abs
  Constant : Constant  Value=0
  Switch : Switch  Criteria=u2 > Threshold  Threshold=5
  Virtual Wall Logic : Outport
  wires:
  Position Error/1 -> Abs/1
  Constant/1 -> Switch/3
  Abs/1 -> Switch/1, Switch/2
  Switch/1 -> Virtual Wall Logic/1

== matlab function HL_control_pos_FFforce_RC_WirtualWall_Sync/From HMI Coord.s/Transform L Hip to HMI Coord.s/RawRef ==
  data: pos output; vel output; pos input; vel input; force input; force output
function [pos, vel, force]  = rotate2HMIcoords(pos, vel, force)
r = -0.264836 + pi;
RzT = [cos(r) -sin(r) 0;
       sin(r)  cos(r) 0;
         0        0   1]';

r = pi;
RxT = [1   0       0;
       0 cos(r) -sin(r);
       0 sin(r)  cos(r)]';

xy = RzT * (RxT * [force(1:2) pos(1:2) vel(1:2); 1 1 1]);

force(1:2) = xy(1:2, 1);
force(3) = -force(3);

pos(1:2) = xy(1:2, 2);
pos(3) = -pos(3);

vel(1:2) = xy(1:2, 3);
vel(3) = -vel(3);

== matlab function HL_control_pos_FFforce_RC_WirtualWall_Sync/To HMI Coord.s/R Leg/pos_vel ==
  data: pos input; pos output; vel input; vel output
function [pos, vel] = rotate2HMIcoords(pos, vel)
r = 0.254574 + pi;
Rz = [cos(r) -sin(r) 0;
      sin(r)  cos(r) 0;
        0        0   1];

xy = Rz * [pos(1:2) vel(1:2); 1 1];

pos(1:2) = xy(1:2, 1);
vel(1:2) = xy(1:2, 2);

== matlab function HL_control_pos_FFforce_RC_WirtualWall_Sync/To HMI Coord.s/R Leg/FTproc ==
  data: theta input; FT input; FT output; massFTr data_store_memory; biasFTr data_store_memory; eccentFTr data_store_memory
function FT = transformFT(theta, FT)

global massFTr biasFTr eccentFTr;

FT = FT - biasFTr.* ones(6, length(theta))...
        - massFTr * [-sin(theta); -cos(theta); zeros(1, length(theta));
                     cos(theta) * eccentFTr(1);
                    -sin(theta) * eccentFTr(1);
                  (eccentFTr(2) * sin(theta) - eccentFTr(3) * cos(theta))];

== matlab function HL_control_pos_FFforce_RC_WirtualWall_Sync/To HMI Coord.s/L Leg/pos_vel ==
  data: pos input; pos output; vel input; vel output
function [pos, vel] = rotate2HMIcoords(pos, vel)
r = -0.264836 + pi;
Rz = [cos(r) -sin(r) 0;
      sin(r)  cos(r) 0;
        0        0   1];

r = pi;
Rx = [ 1   0       0;
       0 cos(r) -sin(r);
       0 sin(r)  cos(r)];

xy = Rx * (Rz * [pos(1:2) vel(1:2); 1 1]);

pos(1:2) = xy(1:2, 1);
vel(1:2) = xy(1:2, 2);
pos(3) = -pos(3);
vel(3) = -vel(3);

== matlab function HL_control_pos_FFforce_RC_WirtualWall_Sync/From HMI Coord.s/Transform R Hip to HMI Coord.s/RawRef ==
  data: pos output; vel output; pos input; vel input; force input; force output
function [pos, vel, force] = rotate2HMIcoords(pos, vel, force)
r = 0.254574 + pi;
RzT = [cos(r) -sin(r) 0;
       sin(r)  cos(r) 0;
        0        0    1]';

xy = RzT * [force(1:2) pos(1:2) vel(1:2); 1 1 1];

force(1:2) = xy(1:2, 1);
pos(1:2) = xy(1:2, 2);
vel(1:2) = xy(1:2, 3);

== stateflow chart HL_control_pos_FFforce_RC_WirtualWall_Sync/High-Level Controller/Reference Generator ==
  settings: sampleTime=0.001
  state SystemON
    entry:
    Pgain = 0;
    Dgain = 0;
    exit:
    Pgain = 0;
    Dgain = 0;
    state setControl1(c) [function]
    state ForceTrajectoryGeneretor
      entry:
      setControl1(48);
      Pgain = 0; Dgain = 0;
      state DataHandling [parallel]
        settings: executionOrder=1
        state ReadData
          hip_torque = read_data();
          state force = read_data [function]
        state Init
          % Wait until new data arrives...
        state Wait4data
        SystemON.ForceTrajectoryGeneretor.DataHandling.Init -> ReadData
        (default) -> SystemON.ForceTrajectoryGeneretor.DataHandling.Init
        ReadData -> Wait4data
      state force = getCustomTrajectory [function] [commented out]
      state Right [parallel]
        settings: executionOrder=2
        state SetRightReference
          entry, during:
          ifr = ifr + 1;
          ref.right.force.Tz = resample_profile(hip_torque, ifr, gait.period)
          exit:
          ref.right.force.Tz = resample_profile(hip_torque, ifr, gait.period)
          ifr = 0;
        state Init
          ifr = 0
          ref.right = setForceBus(...
          ref.right, [0 0 0]);
        (default) -> SystemON.ForceTrajectoryGeneretor.Right.Init
        SystemON.ForceTrajectoryGeneretor.Right.Init -> SetRightReference : [gait.heelstriked.right]
        SetRightReference -> SetRightReference : [gait.heelstriked.right]
      state Left [parallel]
        settings: executionOrder=3
        state SetLeftReference
          entry, during:
          ifl = ifl + 1;
          ref.left.force.Tz = resample_profile(hip_torque, ifl, gait.period)
          exit:
          ref.left.force.Tz = resample_profile(hip_torque, ifl, gait.period)
          ifl = 0;
        state Init
          ifl = 0;
          ref.left = setForceBus(...
          ref.left, [0 0 0]);
        (default) -> SystemON.ForceTrajectoryGeneretor.Left.Init
        SystemON.ForceTrajectoryGeneretor.Left.Init -> SetLeftReference : [gait.heelstriked.left]
        SetLeftReference -> SetLeftReference : [gait.heelstriked.left]
    state Idle
    state MotionTrajectoryGenerator
      entry:
      Pgain = 1; Dgain = 1;
      exit:
      Pgain = 0; Dgain = 0;
      state Calibration
        entry:
        % Set the most smooth filter.
        setControl1(128);
        cal_ref = read_data();
        state Measuring
          entry, during:
          ic = ic + 1;
          ref.right = setMotionBus(ref.right,...
          [0 0 cal_ref(ic, 1)],...
          [0 0 cal_ref(ic, 2)]);
          ref.left = setMotionBus(ref.left,...
          [0 0 cal_ref(ic, 1)],...
          [0 0 cal_ref(ic, 2)]);
          exit:
          icp = icp + 1;
          cal_ft = readFTval(FT, cal_ft, icp);
          cal_mot = readMotVal(mot, cal_mot, icp);
        state Esimating
          calibrate_mass(cal_ft, cal_mot);
        state Init
          ic = 0;
          icp = 0;
          cal_ft = zeros(6, 20, 2);
          cal_mot = zeros(3, 20, 2);
        state Moving
          ic = ic + 1;
          ref.right = setMotionBus(ref.right,...
          [0 0 cal_ref(ic, 1)],...
          [0 0 cal_ref(ic, 2)]);
          ref.left = setMotionBus(ref.left,...
          [0 0 cal_ref(ic, 1)],...
          [0 0 cal_ref(ic, 2)]);
        state cmot = read_data [function]
        Measuring -> Esimating [order 1] : [ic == 58000]
        (default) -> SystemON.MotionTrajectoryGenerator.Calibration.Init
        Measuring -> Moving [order 2] : after(1.7, sec)
        SystemON.MotionTrajectoryGenerator.Calibration.Init -> Measuring
        Moving -> Measuring : after(1.3, sec)
      state Homing
        entry:
        ref.right = setMotionBus(ref.right,...
        [0 0 0],...
        [0 0 0]);
        ref.left = setMotionBus(ref.left,...
        [0 0 0],...
        [0 0 0]);
      state [pos, vel] = testTrajectory [function] [commented out]
      (junction 562) -> Calibration [order 2] : [MODE == 1]
      (junction 562) -> Homing [order 1] : [MODE == 0]
    SystemON -> (junction 549) [order 1] : [hasChanged(MODE)]
    (default) -> (junction 549)
    (junction 549) -> ForceTrajectoryGeneretor [order 1] : [MODE == 2]
    (junction 549) -> (junction 567) [order 2]
    (junction 567) -> Idle [order 2]
    (junction 567) -> (junction 562) [order 1]
    Esimating -> ForceTrajectoryGeneretor
  state Init
    entry:
    ref.right.pos.x = 0; ref.left.pos.x = 0;
    ref.right.pos.y = 0; ref.left.pos.y = 0;
    ref.right.pos.theta = 0; ref.left.pos.theta = 0;
    ref.right.vel.vx = 0; ref.left.vel.vx = 0;
    ref.right.vel.vy = 0; ref.left.vel.vy = 0;
    ref.right.vel.omega = 0; ref.left.vel.omega = 0;
    ref.right.force.Fx = 0; ref.left.force.Fx = 0;
    ref.right.force.Fy = 0; ref.left.force.Fy = 0;
    ref.right.force.Tz = 0; ref.left.force.Tz = 0;
  state SystemOFF
  SystemON -> SystemOFF [order 1] : [~sysON]
  Init -> SystemOFF
  (default) -> Init
  SystemOFF -> SystemON : [sysON]
  data: c function_input double size=1; force function_output; norm_profile function_input; ti function_input; force function_output; period function_input; force function_output double size=1; bus function_input; force function_input; bus function_output; cft function_input; cmot function_input; ThighBus function_input; pts function_output; pts function_input; i function_input; AllMotBus function_input; pts function_output; pts function_input; i function_input; cmot function_output; pos function_output double size=1; vel function_output double size=1; bus function_input; pos function_input; bus function_output; vel function_input; sysON input boolean size=1; ref output Bus: AllRef size=1; hip_torque local double size=60000; ifr local double size=1; ifl local double size=1; Dgain data_store_memory; Pgain data_store_memory; cal_ref local double size=[60000 2]; ic local double size=1; FT input Bus: ThighForces size=1; icp local double size=1; cal_ft local double size=[6 20 2]; mot input Bus: AllMotOut size=1; cal_mot local double size=[3 20 2]; massFTr data_store_memory; massFTl data_store_memory; biasFTr data_store_memory; biasFTl data_store_memory; eccentFTr data_store_memory; eccentFTl data_store_memory; gait input Bus: Gait size=1; MODE input double size=1
  function force = resample_profile(norm_profile, ti, period):
    | function force = resample_profile(norm_profile, ti, period)
    | 
    | period = round(period * 1000);
    | if period == 0 || ti >= period
    |     force = 0;
    | else
    |     t = ti * 1000/period;
    | 
    |     tl = floor(t);
    |     th = ceil(t);
    | 
    |     force = (norm_profile(th+1, 1) - norm_profile(tl+1, 1)) * (t - tl)...
    |         + norm_profile(tl+1, 1);
    | end
  function bus = setForceBus(bus, force):
    | function bus = setForceBus(bus, force)
    | bus.force.Fx = force(1);
    | bus.force.Fy = force(2);
    | bus.force.Tz = force(3);
  function calibrate_mass(cft, cmot):
    | function calibrate_mass(cft, cmot)
    | %% DEFINE MEASURED AND UNKNOWN VARIABLES
    | global massFTr biasFTr eccentFTr massFTl biasFTl eccentFTl;
    | % Partition the collected data according to the sides.
    | rtheta = cmot(3, :, 1)';
    | ltheta = cmot(3, :, 2)';
    | rft = cft(:, :, 1)';
    | lft = cft(:, :, 2)';
    | 
    | %% CALIBRATE THE RIGHT SIDE
    | A = [ones(length(rtheta), 1) sin(rtheta) cos(rtheta)];
    | w = permute(repmat([ones(6, 1) [-eye(2); 0 0; 0 1; -1 0; 1 -1]],...
    |                    [1 1 length(rtheta)]), [3 2 1]);
    | x = zeros(3, 6);
    | for i = 1:6
    |     x(:,i) = (A .* w(:,:,i)) \ rft(:,i);
    | end
    | 
    | massFTr = mean([x(2,1) x(3,2)]);
    | biasFTr = x(1,:)';
    | eccentFTr = [mean([x(3,4)/x(3,2) x(2,5)/x(2,1)]);
    |              x(2,6)/x(2,1);
    |              x(3,6)/x(3,2)];
    | 
    | %% CALIBRATE THE LEFT SIDE
    | A = [ones(length(ltheta), 1) sin(ltheta) cos(ltheta)];
    | w = permute(repmat([ones(6, 1) [-eye(2); 0 0; 0 1; -1 0; 1 -1]],...
    |                    [1 1 length(ltheta)]), [3 2 1]);
    | x = zeros(3, 6);
    | for i = 1:6
    |     x(:,i) = (A .* w(:,:,i)) \ lft(:,i);
    | end
    | 
    | massFTl = mean([x(2,1) x(3,2)]);
    | biasFTl = x(1,:)';
    | eccentFTl = [mean([x(3,4)/x(3,2) x(2,5)/x(2,1)]);
    |              x(2,6)/x(2,1);
    |              x(3,6)/x(3,2)];
  function pts = readFTval(ThighBus, pts, i):
    | function pts = readFTval(ThighBus, pts, i)
    | 
    | pts(:, i, 1) = [ThighBus.right.Fx;
    |                 ThighBus.right.Fy;
    |                 ThighBus.right.Fz;
    |                 ThighBus.right.Tx;
    |                 ThighBus.right.Ty;
    |                 ThighBus.right.Tz];
    | 
    | pts(:, i, 2) = [ThighBus.left.Fx;
    |                 ThighBus.left.Fy;
    |                 ThighBus.left.Fz;
    |                 ThighBus.left.Tx;
    |                 ThighBus.left.Ty;
    |                 ThighBus.left.Tz];
  function pts = readMotVal(AllMotBus, pts, i):
    | function pts = readMotVal(AllMotBus, pts, i)
    | 
    | pts(:, i, 1) = [AllMotBus.right.pos.x;
    |                 AllMotBus.right.pos.y;
    |                 AllMotBus.right.pos.theta];
    | 
    | pts(:, i, 2) = [AllMotBus.left.pos.x;
    |                 AllMotBus.left.pos.y;
    |                 AllMotBus.left.pos.theta];
  function bus = setMotionBus(bus, pos, vel):
    | function bus = setMotionBus(bus, pos, vel)
    | bus.pos.x = pos(1);
    | bus.pos.y = pos(2);
    | bus.pos.theta = pos(3);
    | 
    | bus.vel.vx = vel(1);
    | bus.vel.vy = vel(2);
    | bus.vel.omega = vel(3);

== matlab function HL_control_pos_FFforce_RC_WirtualWall_Sync/To HMI Coord.s/L Leg/FTproc ==
  data: theta input; FT input; FT output; massFTl data_store_memory; biasFTl data_store_memory; eccentFTl data_store_memory
function FT = transformFT(theta, FT)

global massFTl biasFTl eccentFTl;

FT(1:3,:) = roty(180) * FT(1:3,:);
FT(4:6,:) = roty(180) * FT(4:6,:);

FT = FT - biasFTl.* ones(6, length(theta))...
        - massFTl * [-sin(theta); -cos(theta); zeros(1, length(theta));
                     cos(theta) * eccentFTl(1);
                    -sin(theta) * eccentFTl(1);
                  (eccentFTl(2) * sin(theta) - eccentFTl(3) * cos(theta))];
